simulink model "eventcountcomp_ref"  (Simulink 5.0)
settings: Solver=FixedStepDiscrete  StartTime=0.0  StopTime=30  RelTol=1e-3
PostLoadFcn:
  | set_param(gcs,'SimulationCommand','Update')
libraries: dspsrcs4 x2, dspswit3 x1
settings Model: RequirementInfo=9  Creator=ckamachi  LastModifiedBy=ckamachi  ExtModeTrigMode=oneshot  ExtModeArmWhenConnect=off  LimitDataPoints=off  BlockReductionOpt=off  BooleanDataType=off

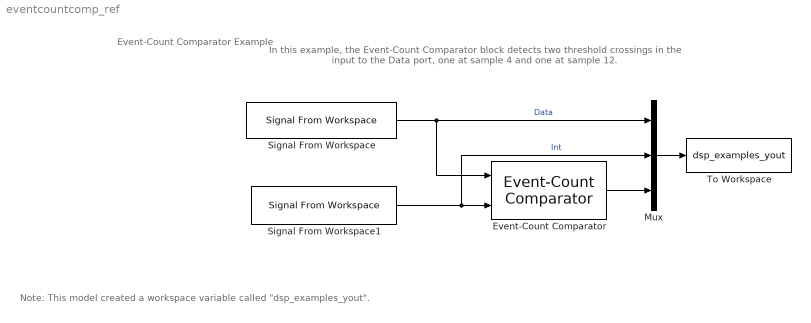
== system eventcountcomp_ref ==
  note: Event-Count Comparator Example
  note: In this example, the Event-Count Comparator block detects two threshold
      | crossings in the input to the Data port, one at sample 4 and one at sample 12.
  note: Note: This model created a workspace variable called "dsp_examples_yout".
  Event-Count Comparator : dspswit3/Event-Count Comparator  Threshold=3
  Mux : Mux  Inputs=3
  Signal From Workspace : dspsrcs4/Signal From Workspace  X=[0 1 2 3 4 5 0 0 0 5 4 3 2 1 0]  Ts=1  nsamps=1  OutputAfterFinalValue=Setting to zero
  Signal From Workspace1 : dspsrcs4/Signal From Workspace  X=[0 1 1 1 1 1 0 0 1 1 1 1 1 1 0]  Ts=1  nsamps=1  OutputAfterFinalValue=Setting to zero
  To Workspace : ToWorkspace  VariableName=dsp_examples_yout  SampleTime=-1  SaveFormat=Array
  wires:
  Signal From Workspace/1 -> Mux/1, Event-Count Comparator/1  "Data"
  Signal From Workspace1/1 -> Mux/2, Event-Count Comparator/2  "Int"
  Mux/1 -> To Workspace/1
  Event-Count Comparator/1 -> Mux/3
